simulink model "Model_Te05_R2020b"  (R2020b)
settings: Solver=FixedStepAuto  StartTime=0.0  StopTime=25  FixedStep=0.5  RelTol=1e-3
undefined symbols (not defined in the file or in its folder): serial
libraries: instrumentlib x3
settings Model: Creator=berci  LastModifiedBy=Berciu Alexandru
settings DataIOCC: ReturnWorkspaceOutputs=off
settings DebuggingCC: ArithmeticOperatorsInVariantConditions=warning
settings SFSimCC: SimUseLocalCustomCode=off  CustomCodeUndefinedFunction=UseInterfaceOnly
settings RTWCC: RTWUseLocalCustomCode=off

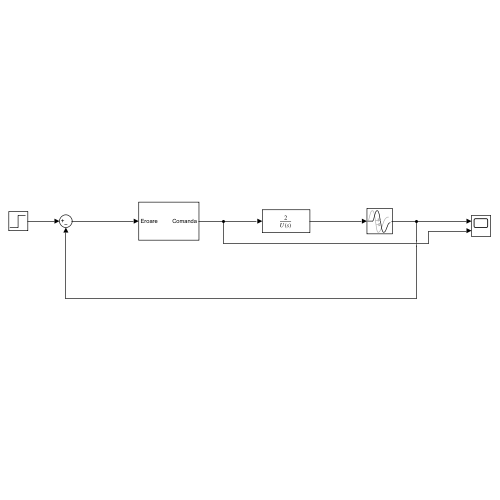
[thumbnail: Simulink's stored preview of the top-level diagram]
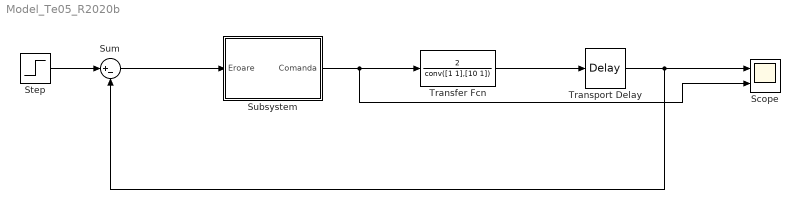
== system Model_Te05_R2020b ==
  Scope : Scope  NumInputPorts=2
  Step : Step  Time=0  SampleTime=0.5
  Subsystem : Subsystem
  Sum : Sum  Inputs=|+-
  Transfer Fcn : TransferFcn  Numerator=[2]  Denominator=conv([1 1],[10 1])
  Transport Delay : TransportDelay
  wires:
  Transport Delay/1 -> Sum/2, Scope/1
  Transfer Fcn/1 -> Transport Delay/1
  Subsystem/1(Comanda) -> Scope/2, Transfer Fcn/1
  Sum/1 -> Subsystem/1(Eroare)
  Step/1 -> Sum/1

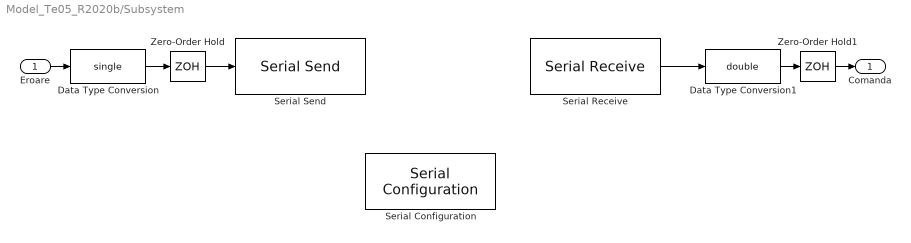
== system Model_Te05_R2020b/Subsystem ==
  Eroare : Inport
  Data Type Conversion : DataTypeConversion  OutDataTypeStr=single
  Data Type Conversion1 : DataTypeConversion  OutDataTypeStr=double
  Serial Configuration : instrumentlib/Serial Configuration  Priority=-200000  ObjConstructor=serial('COM3');  ComPortMenu=COM3  ComPort=COM3  BaudRate=9600  DataBits=8  Parity=none  StopBits=1  ByteOrder=LittleEndian  FlowControl=none  Timeout=10
  Serial Receive : instrumentlib/Serial Receive  ObjConstructor=serial('COM3');  ComPortMenu=COM3  ComPort=COM3  DataType=single  DataSize=[1 1]  Terminator=<none>  EnableBlockingMode=on  ActionDataUnavailable=Output last received value  CustomValue=0  SampleTime=0.5
  Serial Send : instrumentlib/Serial Send  ObjConstructor=serial('COM3');  ComPortMenu=COM3  ComPort=COM3  Terminator=<none>  EnableBlockingMode=on
  Zero-Order Hold : ZeroOrderHold  SampleTime=0.5
  Zero-Order Hold1 : ZeroOrderHold  SampleTime=0.5
  Comanda : Outport  VectorParamsAs1DForOutWhenUnconnected=off
  wires:
  Eroare/1 -> Data Type Conversion/1
  Zero-Order Hold1/1 -> Comanda/1
  Data Type Conversion1/1 -> Zero-Order Hold1/1
  Serial Receive/1 -> Data Type Conversion1/1
  Zero-Order Hold/1 -> Serial Send/1
  Data Type Conversion/1 -> Zero-Order Hold/1
